simulink model "ThdRwLtStCalib"  (R2024b)
settings: Solver=FixedStepDiscrete  StartTime=0.0  StopTime=10.0  FixedStep=0.01  RelTol=1e-3
model workspace (MAT data in the model file):
  KeSMSwAcsMd6ThdRwLtStBkReclnUpwdDnwdPosMax_Val = Simulink.Parameter
  KeSMSwAcsMd6ThdRwLtStBkReclnUpwdDnwdPosMax_Val.Value = 0
  KeSMSwAcsMd6ThdRwLtStBkReclnUpwdDnwdPosMax_Val.Complexity = 'real'
  KeSMSwAcsMd6ThdRwLtStBkReclnUpwdDnwdPosMax_Val.Dimensions = [1 1]
  KeSMSwAcsMd6ThdRwLtStBkReclnUpwdDnwdPosMax_Val.DataType = 'uint16'
  KeSMSwAcsMd6ThdRwLtStBkReclnUpwdDnwdPosMin_Val = Simulink.Parameter
  KeSMSwAcsMd6ThdRwLtStBkReclnUpwdDnwdPosMin_Val.Value = 0
  KeSMSwAcsMd6ThdRwLtStBkReclnUpwdDnwdPosMin_Val.Complexity = 'real'
  KeSMSwAcsMd6ThdRwLtStBkReclnUpwdDnwdPosMin_Val.Dimensions = [1 1]
  KeSMSwAcsMd6ThdRwLtStBkReclnUpwdDnwdPosMin_Val.DataType = 'uint16'
  KeSMSwAcsMd6ThdRwLtStBkReclnUpwdDnwdPos_Val = Simulink.Parameter
  KeSMSwAcsMd6ThdRwLtStBkReclnUpwdDnwdPos_Val.Value = 0
  KeSMSwAcsMd6ThdRwLtStBkReclnUpwdDnwdPos_Val.Complexity = 'real'
  KeSMSwAcsMd6ThdRwLtStBkReclnUpwdDnwdPos_Val.Dimensions = [1 1]
  KeSMSwAcsMd6ThdRwLtStBkReclnUpwdDnwdPos_Val.DataType = 'uint16'
  KeSMSwAcsMd6ThdRwLtStCshnFldUpwdDnwdPosMax_Val = Simulink.Parameter
  KeSMSwAcsMd6ThdRwLtStCshnFldUpwdDnwdPosMax_Val.Value = 0
  KeSMSwAcsMd6ThdRwLtStCshnFldUpwdDnwdPosMax_Val.Complexity = 'real'
  KeSMSwAcsMd6ThdRwLtStCshnFldUpwdDnwdPosMax_Val.Dimensions = [1 1]
  KeSMSwAcsMd6ThdRwLtStCshnFldUpwdDnwdPosMax_Val.DataType = 'uint16'
  KeSMSwAcsMd6ThdRwLtStCshnFldUpwdDnwdPosMin_Val = Simulink.Parameter
  KeSMSwAcsMd6ThdRwLtStCshnFldUpwdDnwdPosMin_Val.Value = 0
  KeSMSwAcsMd6ThdRwLtStCshnFldUpwdDnwdPosMin_Val.Complexity = 'real'
  KeSMSwAcsMd6ThdRwLtStCshnFldUpwdDnwdPosMin_Val.Dimensions = [1 1]
  KeSMSwAcsMd6ThdRwLtStCshnFldUpwdDnwdPosMin_Val.DataType = 'uint16'
  KeSMSwAcsMd6ThdRwLtStCshnFldUpwdDnwdPos_Val = Simulink.Parameter
  KeSMSwAcsMd6ThdRwLtStCshnFldUpwdDnwdPos_Val.Value = 0
  KeSMSwAcsMd6ThdRwLtStCshnFldUpwdDnwdPos_Val.Complexity = 'real'
  KeSMSwAcsMd6ThdRwLtStCshnFldUpwdDnwdPos_Val.Dimensions = [1 1]
  KeSMSwAcsMd6ThdRwLtStCshnFldUpwdDnwdPos_Val.DataType = 'uint16'
  KeSMSwAcsMd6ThdRwLtStFrwdBkwdPosMax_Val = Simulink.Parameter
  KeSMSwAcsMd6ThdRwLtStFrwdBkwdPosMax_Val.Value = 0
  KeSMSwAcsMd6ThdRwLtStFrwdBkwdPosMax_Val.Complexity = 'real'
  KeSMSwAcsMd6ThdRwLtStFrwdBkwdPosMax_Val.Dimensions = [1 1]
  KeSMSwAcsMd6ThdRwLtStFrwdBkwdPosMax_Val.DataType = 'uint16'
  KeSMSwAcsMd6ThdRwLtStFrwdBkwdPosMin_Val = Simulink.Parameter
  KeSMSwAcsMd6ThdRwLtStFrwdBkwdPosMin_Val.Value = 0
  KeSMSwAcsMd6ThdRwLtStFrwdBkwdPosMin_Val.Complexity = 'real'
  KeSMSwAcsMd6ThdRwLtStFrwdBkwdPosMin_Val.Dimensions = [1 1]
  KeSMSwAcsMd6ThdRwLtStFrwdBkwdPosMin_Val.DataType = 'uint16'
  KeSMSwAcsMd6ThdRwLtStFrwdBkwdPos_Val = Simulink.Parameter
  KeSMSwAcsMd6ThdRwLtStFrwdBkwdPos_Val.Value = 0
  KeSMSwAcsMd6ThdRwLtStFrwdBkwdPos_Val.Complexity = 'real'
  KeSMSwAcsMd6ThdRwLtStFrwdBkwdPos_Val.Dimensions = [1 1]
  KeSMSwAcsMd6ThdRwLtStFrwdBkwdPos_Val.DataType = 'uint16'
undefined symbols (not defined in the file or in its folder): KeSMSw6sAcsEntryThdRwLtStBkReclnUpwdDnwdPos_Val, KeSMSw6sAcsEntryThdRwLtStBkReclnUpwdDnwdPosMax_Val, KeSMSw6sAcsEntryThdRwLtStBkReclnUpwdDnwdPosMin_Val, KeSMSw6sAcsEntryThdRwLtStCshnFldUpwdDnwdPos_Val, KeSMSw6sAcsEntryThdRwLtStCshnFldUpwdDnwdPosMax_Val, KeSMSw6sAcsEntryThdRwLtStCshnFldUpwdDnwdPosMin_Val, KeSMSw6sAcsEntryThdRwLtStFrwdBkwdPos_Val, KeSMSw6sAcsEntryThdRwLtStFrwdBkwdPosMax_Val, KeSMSw6sAcsEntryThdRwLtStFrwdBkwdPosMin_Val, KeSMSw6SAcsMd56ThdRwLtStBkReclnUpwdDnwdPos_Val, KeSMSw6SAcsMd56ThdRwLtStBkReclnUpwdDnwdPosMax_Val, KeSMSw6SAcsMd56ThdRwLtStBkReclnUpwdDnwdPosMin_Val, KeSMSw6SAcsMd56ThdRwLtStFrwdBkwdPos_Val, KeSMSw6SAcsMd56ThdRwLtStFrwdBkwdPosMax_Val, KeSMSw6SAcsMd56ThdRwLtStFrwdBkwdPosMin_Val, KeSMSw6sFamilyLMdThdRwLtStFrwdBkwdPos_Val, KeSMSw6sFamilyLMdThdRwLtStFrwdBkwdPosMax_Val, KeSMSw6sFamilyLMdThdRwLtStFrwdBkwdPosMin_Val, KeSMSw6sFamilyMdThdRwLtStFrwdBkwdPos_Val, KeSMSw6sFamilyMdThdRwLtStFrwdBkwdPosMax_Val, KeSMSw6sFamilyMdThdRwLtStFrwdBkwdPosMin_Val, KeSMSw6sLugThdRwLtStBkReclnUpwdDnwdPos_Val, KeSMSw6sLugThdRwLtStBkReclnUpwdDnwdPosMax_Val, KeSMSw6sLugThdRwLtStBkReclnUpwdDnwdPosMin_Val, KeSMSw6sLugThdRwLtStCshnFldUpwdDnwdPos_Val, KeSMSw6sLugThdRwLtStCshnFldUpwdDnwdPosMax_Val, KeSMSw6sLugThdRwLtStCshnFldUpwdDnwdPosMin_Val, KeSMSw6sVIPThdRwLtStBkReclnUpwdDnwdPos_Val, KeSMSw6sVIPThdRwLtStBkReclnUpwdDnwdPosMax_Val, KeSMSw6sVIPThdRwLtStBkReclnUpwdDnwdPosMin_Val, KeSMSw6sVIPThdRwLtStFrwdBkwdPos_Val, KeSMSw6sVIPThdRwLtStFrwdBkwdPosMax_Val, KeSMSw6sVIPThdRwLtStFrwdBkwdPosMin_Val, KeSMSwAcsEntryThdRwLtStBkReclnUpwdDnwdPos_Val, KeSMSwAcsEntryThdRwLtStBkReclnUpwdDnwdPosMax_Val, KeSMSwAcsEntryThdRwLtStBkReclnUpwdDnwdPosMin_Val, KeSMSwAcsEntryThdRwLtStCshnFldUpwdDnwdPos_Val, KeSMSwAcsEntryThdRwLtStCshnFldUpwdDnwdPosMax_Val, KeSMSwAcsEntryThdRwLtStCshnFldUpwdDnwdPosMin_Val, KeSMSwAcsEntryThdRwLtStFrwdBkwdPos_Val, KeSMSwAcsEntryThdRwLtStFrwdBkwdPosMax_Val, KeSMSwAcsEntryThdRwLtStFrwdBkwdPosMin_Val, KeSMSwAcsMd32ThdRwLtBkReclnUpwdDnwdPos_Val, KeSMSwAcsMd32ThdRwLtBkReclnUpwdDnwdPosMax_Val, KeSMSwAcsMd32ThdRwLtBkReclnUpwdDnwdPosMin_Val, KeSMSwAcsMd32ThdRwLtFldUpwdDnwdPos_Val, KeSMSwAcsMd32ThdRwLtFldUpwdDnwdPosMax_Val, KeSMSwAcsMd32ThdRwLtFldUpwdDnwdPosMin_Val, KeSMSwAcsMd56ThdRwLtStBkReclnUpwdDnwdPos_Val, KeSMSwAcsMd56ThdRwLtStBkReclnUpwdDnwdPosMax_Val, KeSMSwAcsMd56ThdRwLtStBkReclnUpwdDnwdPosMin_Val, KeSMSwAcsMd56ThdRwLtStCshnFldUpwdDnwdPos_Val, KeSMSwAcsMd56ThdRwLtStCshnFldUpwdDnwdPosMax_Val, KeSMSwAcsMd56ThdRwLtStCshnFldUpwdDnwdPosMin_Val, KeSMSwAcsMd56ThdRwLtStFrwdBkwdPos_Val, KeSMSwAcsMd56ThdRwLtStFrwdBkwdPosMax_Val, KeSMSwAcsMd56ThdRwLtStFrwdBkwdPosMin_Val, KeSMSwAcsMd57ThdRwLtStBkReclnUpwdDnwdPos_Val, KeSMSwAcsMd57ThdRwLtStBkReclnUpwdDnwdPosMax_Val, KeSMSwAcsMd57ThdRwLtStBkReclnUpwdDnwdPosMin_Val ... (+28)
libraries: TrgtPosSelcLib x20
(part 1 of 2)
settings Model: ParameterArgumentNames=KeSMSwAcsMd6ThdRwLtStBkReclnUpwdDnwdPosMax_Val,KeSMSwAcsMd6ThdRwLtStBkReclnUpwdDnwdPosMin_Val,KeSMSwAcsMd6ThdRwLtStBkReclnUpwdDnwdPos_Val,KeSMSwAcsMd6ThdRwLtStCshnFldUpwdDnwdPosMax_Val,KeSMSwAcsMd6ThdRwLtStCshnFldUpwdDnwdPosMin_Val,KeSMSwAcsMd6ThdRwLtStCshnFldUpwdDnwdPos_Val,KeSMSwAcsMd6ThdRwLtStFrwdBkwdPosMax_Val,KeSMSwAcsMd6ThdRwLtStFrwdBkwdPosMin_Val,KeSMSwAcsMd6ThdRwLtStFrwdBkwdPos_Val  Creator=sn2xws  LastModifiedBy=sn55gm
settings Model: ModifiedHistory=|
  | 增加Md57，Md58标定，增加6sBitMask
  | 2025.3.5 V3.9.0 Bug 998429 LUG模式偶发不会往前移动三排，但是报成功
settings SolverCC: AlgebraicLoopSolver=TrustRegion
settings DataIOCC: SaveFormat=StructureWithTime  ReturnWorkspaceOutputs=off
settings OptimizationCC: DefaultParameterBehavior=Inlined  EnhancedBackFolding=on  PassReuseOutputArgsAs=Individual arguments  ZeroExternalMemoryAtStartup=off  ZeroInternalMemoryAtStartup=off  OptimizeBlockOrder=speed  DifferentSizesBufferReuse=on  OptimizationCustomize=off  EfficientTunableParamExpr=on
settings DebuggingCC: ParameterTunabilityLossMsg=error  UnconnectedInputMsg=warning  UnconnectedOutputMsg=warning  UnconnectedLineMsg=warning  ArithmeticOperatorsInVariantConditions=warning
settings ModelReferenceCC: EnableRefExpFcnMdlSchedulingChecks=on
settings SFSimCC: MATLABDynamicMemAlloc=off  CustomCodeUndefinedFunction=UseInterfaceOnly
settings RTWCC: Description=AUTOSAR  SystemTargetFile=autosar.tlc  GenCodeOnly=on  TemplateMakefile=ert_default_tmf  GenerateReport=on  IncludeHyperlinkInReport=on  LaunchReport=on  DataTypeReplacement=CDataTypesFixedWidth  GenerateTraceInfo=on  GenerateTraceReport=on  GenerateTraceReportSl=on  GenerateTraceReportSf=on  GenerateTraceReportEml=on  GPUComputeCapability=3.5
settings CodeAppCC: ForceParamTrailComments=on  IgnoreCustomStorageClasses=off  OperatorAnnotations=on  SimulinkDataObjDesc=on  SFDataObjDesc=on  InsertBlockDesc=on
settings STFCustomTargetCC: TargetLangStandard=C99 (ISO)  MultiwordLength=256  ParMdlRefBuildCompliant=on  CompOptLevelCompliant=on  IncludeMdlTerminateFcn=off  CombineOutputUpdateFcns=on  SuppressErrorStatus=on  ERTCustomFileBanners=on  SupportNonFinite=off  SupportComplex=off  SupportContinuousTime=off  SupportNonInlinedSFcns=off  RemoveResetFunc=on  MATLABClassNameForMDSCustomization=Simulink.SoftwareTarget.ERTCustomization  AutosarCompliant=on  UseToolchainInfoCompliant=on  LookupTableObjectStructAxisOrder=2,1,3,4,...  LUTObjectStructOrderEvenSpacing=Size,Table,Breakpoints  SystemTargetFile=autosar.tlc
settings ERTTargetCC: TargetLangStandard=C99 (ISO)  ConcurrentExecutionCompliant=off  IncludeMdlTerminateFcn=off  SuppressErrorStatus=on  SupportNonFinite=off  SupportComplex=off  ModelStepFunctionPrototypeControlCompliant=off  CPPClassGenCompliant=off  AutosarCompliant=on  LookupTableObjectStructAxisOrder=2,1,3,4,...  LUTObjectStructOrderEvenSpacing=Size,Table,Breakpoints  ERTCustomFileTemplate=example_file_process.tlc  ERTFilePackagingFormat=Compact  BooleanTrueId=TRUE  BooleanFalseId=FALSE  DynamicArrayContainerType=coder::array

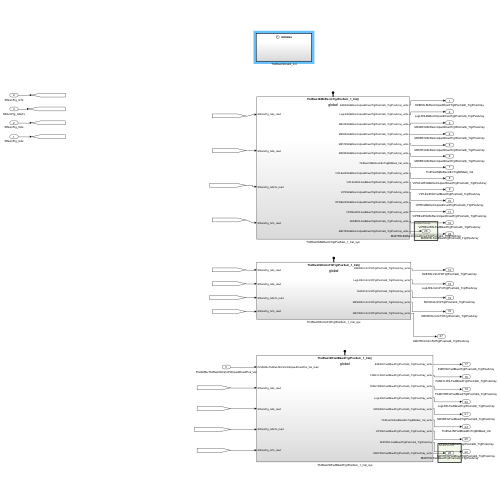
[thumbnail: Simulink's stored preview of the top-level diagram]
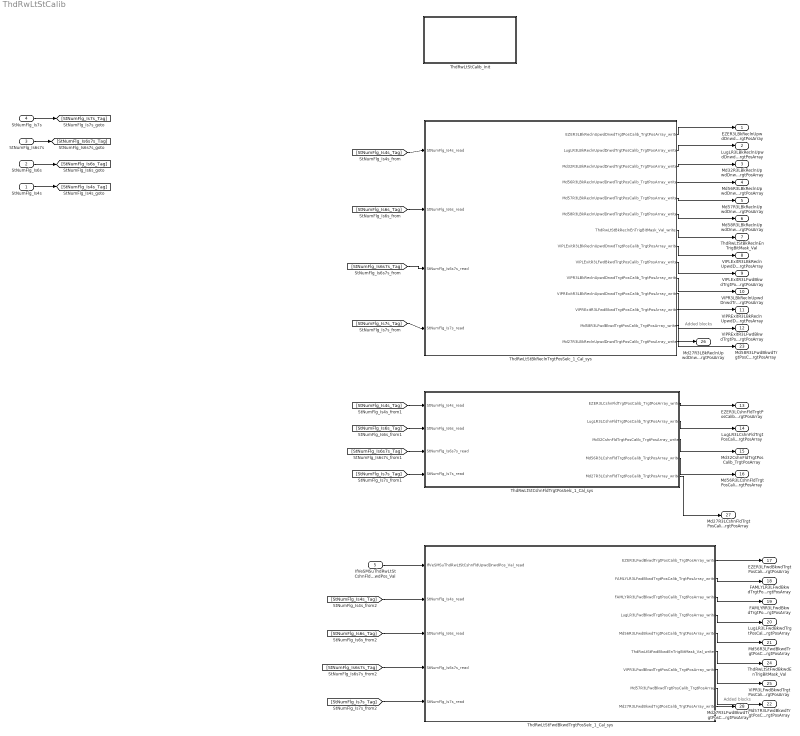
== system ThdRwLtStCalib ==
  note: Added blocks
  note: Added blocks
  StNumFlg_Is4s : Inport  OutDataTypeStr=boolean  PortDimensions=1
  StNumFlg_Is6s : Inport  Port=2  OutDataTypeStr=boolean  PortDimensions=1
  StNumFlg_Is6s7s : Inport  Port=3  OutDataTypeStr=boolean  PortDimensions=1
  StNumFlg_Is7s : Inport  Port=4  OutDataTypeStr=boolean  PortDimensions=1
  IfVeSMSuThdRwLtStCshnFldUpwdDnwdPos_Val : Inport  Port=5  OutDataTypeStr=uint16  PortDimensions=1
  ThdRwLtStBkReclnTrgtPosSelc_1_Cal_sys : Subsystem
  ThdRwLtStCalib_Init : Subsystem
  ThdRwLtStCshnFldTrgtPosSelc_1_Cal_sys : Subsystem
  ThdRwLtStFwdBkwdTrgtPosSelc_1_Cal_sys : Subsystem
  EZER3LBkReclnUpwdDnwdTrgtPosCalib_TrgtPosArray : Outport  Description=|  OutDataTypeStr=uint16  PortDimensions=3  VectorParamsAs1DForOutWhenUnconnected=off
      | 0:Pos
      | 1:Max
      | 2:Min
  LugLR3LBkReclnUpwdDnwdTrgtPosCalib_TrgtPosArray : Outport  Description=|  Port=2  OutDataTypeStr=uint16  PortDimensions=3  VectorParamsAs1DForOutWhenUnconnected=off
      | 0:Pos
      | 1:Max
      | 2:Min
  Md32R3LBkReclnUpwdDnwdTrgtPosCalib_TrgtPosArray : Outport  Description=|  Port=3  OutDataTypeStr=uint16  PortDimensions=3  VectorParamsAs1DForOutWhenUnconnected=off
      | 0:Pos
      | 1:Max
      | 2:Min
  Md56R3LBkReclnUpwdDnwdTrgtPosCalib_TrgtPosArray : Outport  Description=|  Port=4  OutDataTypeStr=uint16  PortDimensions=3  VectorParamsAs1DForOutWhenUnconnected=off
      | 0:Pos
      | 1:Max
      | 2:Min
  Md57R3LBkReclnUpwdDnwdTrgtPosCalib_TrgtPosArray : Outport  Description=|  Port=5  OutDataTypeStr=uint16  PortDimensions=3  VectorParamsAs1DForOutWhenUnconnected=off
      | 0:Pos
      | 1:Max
      | 2:Min
  Md58R3LBkReclnUpwdDnwdTrgtPosCalib_TrgtPosArray : Outport  Description=|  Port=6  OutDataTypeStr=uint16  PortDimensions=3  VectorParamsAs1DForOutWhenUnconnected=off
      | 0:Pos
      | 1:Max
      | 2:Min
  ThdRwLtStBkReclnEnTrigBitMask_Val : Outport  Port=7  OutDataTypeStr=uint32  PortDimensions=1  VectorParamsAs1DForOutWhenUnconnected=off
  VIPLExitR3LBkReclnUpwdDnwdTrgtPosCalib_TrgtPosArray : Outport  Description=|  Port=8  OutDataTypeStr=uint16  PortDimensions=3  VectorParamsAs1DForOutWhenUnconnected=off
      | 0:Pos
      | 1:Max
      | 2:Min
  VIPLExitR3LFwdBkwdTrgtPosCalib_TrgtPosArray : Outport  Description=|  Port=9  OutDataTypeStr=uint16  PortDimensions=3  VectorParamsAs1DForOutWhenUnconnected=off
      | 0:Pos
      | 1:Max
      | 2:Min
  VIPR3LBkReclnUpwdDnwdTrgtPosCalib_TrgtPosArray : Outport  Description=|  Port=10  OutDataTypeStr=uint16  PortDimensions=3  VectorParamsAs1DForOutWhenUnconnected=off
      | 0:Pos
      | 1:Max
      | 2:Min
  VIPRExitR3LBkReclnUpwdDnwdTrgtPosCalib_TrgtPosArray : Outport  Description=|  Port=11  OutDataTypeStr=uint16  PortDimensions=3  VectorParamsAs1DForOutWhenUnconnected=off
      | 0:Pos
      | 1:Max
      | 2:Min
  VIPRExitR3LFwdBkwdTrgtPosCalib_TrgtPosArray : Outport  Description=|  Port=12  OutDataTypeStr=uint16  PortDimensions=3  VectorParamsAs1DForOutWhenUnconnected=off
      | 0:Pos
      | 1:Max
      | 2:Min
  EZER3LCshnFldTrgtPosCalib_TrgtPosArray : Outport  Description=|  Port=13  OutDataTypeStr=uint16  PortDimensions=3  VectorParamsAs1DForOutWhenUnconnected=off
      | 0:Pos
      | 1:Max
      | 2:Min
  LugLR3LCshnFldTrgtPosCalib_TrgtPosArray : Outport  Description=|  Port=14  OutDataTypeStr=uint16  PortDimensions=3  VectorParamsAs1DForOutWhenUnconnected=off
      | 0:Pos
      | 1:Max
      | 2:Min
  Md32CshnFldTrgtPosCalib_TrgtPosArray : Outport  Description=|  Port=15  OutDataTypeStr=uint16  PortDimensions=3  VectorParamsAs1DForOutWhenUnconnected=off
      | 0:Pos
      | 1:Max
      | 2:Min
  Md56R3LCshnFldTrgtPosCalib_TrgtPosArray : Outport  Description=|  Port=16  OutDataTypeStr=uint16  PortDimensions=3  VectorParamsAs1DForOutWhenUnconnected=off
      | 0:Pos
      | 1:Max
      | 2:Min
  EZER3LFwdBkwdTrgtPosCalib_TrgtPosArray : Outport  Description=|  Port=17  OutDataTypeStr=uint16  PortDimensions=3  VectorParamsAs1DForOutWhenUnconnected=off
      | 0:Pos
      | 1:Max
      | 2:Min
  FAMLYLR3LFwdBkwdTrgtPosCalib_TrgtPosArray : Outport  Description=|  Port=18  OutDataTypeStr=uint16  PortDimensions=3  VectorParamsAs1DForOutWhenUnconnected=off
      | 0:Pos
      | 1:Max
      | 2:Min
  FAMLYRR3LFwdBkwdTrgtPosCalib_TrgtPosArray : Outport  Description=|  Port=19  OutDataTypeStr=uint16  PortDimensions=3  VectorParamsAs1DForOutWhenUnconnected=off
      | 0:Pos
      | 1:Max
      | 2:Min
  LugLR3LFwdBkwdTrgtPosCalib_TrgtPosArray : Outport  Description=|  Port=20  OutDataTypeStr=uint16  PortDimensions=3  VectorParamsAs1DForOutWhenUnconnected=off
      | 0:Pos
      | 1:Max
      | 2:Min
  Md56R3LFwdBkwdTrgtPosCalib_TrgtPosArray : Outport  Description=|  Port=21  OutDataTypeStr=uint16  PortDimensions=3  VectorParamsAs1DForOutWhenUnconnected=off
      | 0:Pos
      | 1:Max
      | 2:Min
  Md57R3LFwdBkwdTrgtPosCalib_TrgtPosArray : Outport  Description=|  Port=22  OutDataTypeStr=uint16  PortDimensions=3  VectorParamsAs1DForOutWhenUnconnected=off
      | 0:Pos
      | 1:Max
      | 2:Min
  Md58R3LFwdBkwdTrgtPosCalib_TrgtPosArray : Outport  Description=|  Port=23  OutDataTypeStr=uint16  PortDimensions=3  VectorParamsAs1DForOutWhenUnconnected=off
      | 0:Pos
      | 1:Max
      | 2:Min
  ThdRwLtStFwdBkwdEnTrigBitMask_Val : Outport  Port=24  OutDataTypeStr=uint32  PortDimensions=1  VectorParamsAs1DForOutWhenUnconnected=off
  VIPR3LFwdBkwdTrgtPosCalib_TrgtPosArray : Outport  Description=|  Port=25  OutDataTypeStr=uint16  PortDimensions=3  VectorParamsAs1DForOutWhenUnconnected=off
      | 0:Pos
      | 1:Max
      | 2:Min
  Md27R3LBkReclnUpwdDnwdTrgtPosCalib_TrgtPosArray : Outport  Description=|  Port=26  OutDataTypeStr=uint16  PortDimensions=3  VectorParamsAs1DForOutWhenUnconnected=off
      | 0:Pos
      | 1:Max
      | 2:Min
  Md27R3LCshnFldTrgtPosCalib_TrgtPosArray : Outport  Description=|  Port=27  OutDataTypeStr=uint16  PortDimensions=3  VectorParamsAs1DForOutWhenUnconnected=off
      | 0:Pos
      | 1:Max
      | 2:Min
  Md27R3LFwdBkwdTrgtPosCalib_TrgtPosArray : Outport  Description=|  Port=28  OutDataTypeStr=uint16  PortDimensions=3  VectorParamsAs1DForOutWhenUnconnected=off
      | 0:Pos
      | 1:Max
      | 2:Min
  wires:
  ThdRwLtStBkReclnTrgtPosSelc_1_Cal_sys/1(EZER3LBkReclnUpwdDnwdTrgtPosCalib_TrgtPosArray_write) -> EZER3LBkReclnUpwdDnwdTrgtPosCalib_TrgtPosArray/1
  ThdRwLtStBkReclnTrgtPosSelc_1_Cal_sys/2(LugLR3LBkReclnUpwdDnwdTrgtPosCalib_TrgtPosArray_write) -> LugLR3LBkReclnUpwdDnwdTrgtPosCalib_TrgtPosArray/1
  ThdRwLtStBkReclnTrgtPosSelc_1_Cal_sys/3(Md32R3LBkReclnUpwdDnwdTrgtPosCalib_TrgtPosArray_write) -> Md32R3LBkReclnUpwdDnwdTrgtPosCalib_TrgtPosArray/1
  ThdRwLtStBkReclnTrgtPosSelc_1_Cal_sys/4(Md56R3LBkReclnUpwdDnwdTrgtPosCalib_TrgtPosArray_write) -> Md56R3LBkReclnUpwdDnwdTrgtPosCalib_TrgtPosArray/1
  ThdRwLtStBkReclnTrgtPosSelc_1_Cal_sys/5(Md57R3LBkReclnUpwdDnwdTrgtPosCalib_TrgtPosArray_write) -> Md57R3LBkReclnUpwdDnwdTrgtPosCalib_TrgtPosArray/1
  ThdRwLtStBkReclnTrgtPosSelc_1_Cal_sys/6(Md58R3LBkReclnUpwdDnwdTrgtPosCalib_TrgtPosArray_write) -> Md58R3LBkReclnUpwdDnwdTrgtPosCalib_TrgtPosArray/1
  ThdRwLtStBkReclnTrgtPosSelc_1_Cal_sys/7(ThdRwLtStBkReclnEnTrigBitMask_Val_write) -> ThdRwLtStBkReclnEnTrigBitMask_Val/1
  ThdRwLtStBkReclnTrgtPosSelc_1_Cal_sys/8(VIPLExitR3LBkReclnUpwdDnwdTrgtPosCalib_TrgtPosArray_write) -> VIPLExitR3LBkReclnUpwdDnwdTrgtPosCalib_TrgtPosArray/1
  ThdRwLtStBkReclnTrgtPosSelc_1_Cal_sys/9(VIPLExitR3LFwdBkwdTrgtPosCalib_TrgtPosArray_write) -> VIPLExitR3LFwdBkwdTrgtPosCalib_TrgtPosArray/1
  ThdRwLtStBkReclnTrgtPosSelc_1_Cal_sys/10(VIPR3LBkReclnUpwdDnwdTrgtPosCalib_TrgtPosArray_write) -> VIPR3LBkReclnUpwdDnwdTrgtPosCalib_TrgtPosArray/1
  ThdRwLtStBkReclnTrgtPosSelc_1_Cal_sys/11(VIPRExitR3LBkReclnUpwdDnwdTrgtPosCalib_TrgtPosArray_write) -> VIPRExitR3LBkReclnUpwdDnwdTrgtPosCalib_TrgtPosArray/1
  ThdRwLtStBkReclnTrgtPosSelc_1_Cal_sys/12(VIPRExitR3LFwdBkwdTrgtPosCalib_TrgtPosArray_write) -> VIPRExitR3LFwdBkwdTrgtPosCalib_TrgtPosArray/1
  ThdRwLtStCshnFldTrgtPosSelc_1_Cal_sys/1(EZER3LCshnFldTrgtPosCalib_TrgtPosArray_write) -> EZER3LCshnFldTrgtPosCalib_TrgtPosArray/1
  ThdRwLtStCshnFldTrgtPosSelc_1_Cal_sys/2(LugLR3LCshnFldTrgtPosCalib_TrgtPosArray_write) -> LugLR3LCshnFldTrgtPosCalib_TrgtPosArray/1
  ThdRwLtStCshnFldTrgtPosSelc_1_Cal_sys/3(Md32CshnFldTrgtPosCalib_TrgtPosArray_write) -> Md32CshnFldTrgtPosCalib_TrgtPosArray/1
  ThdRwLtStCshnFldTrgtPosSelc_1_Cal_sys/4(Md56R3LCshnFldTrgtPosCalib_TrgtPosArray_write) -> Md56R3LCshnFldTrgtPosCalib_TrgtPosArray/1
  IfVeSMSuThdRwLtStCshnFldUpwdDnwdPos_Val/1 -> ThdRwLtStFwdBkwdTrgtPosSelc_1_Cal_sys/1(IfVeSMSuThdRwLtStCshnFldUpwdDnwdPos_Val_read)
  ThdRwLtStFwdBkwdTrgtPosSelc_1_Cal_sys/1(EZER3LFwdBkwdTrgtPosCalib_TrgtPosArray_write) -> EZER3LFwdBkwdTrgtPosCalib_TrgtPosArray/1
  ThdRwLtStFwdBkwdTrgtPosSelc_1_Cal_sys/2(FAMLYLR3LFwdBkwdTrgtPosCalib_TrgtPosArray_write) -> FAMLYLR3LFwdBkwdTrgtPosCalib_TrgtPosArray/1
  ThdRwLtStFwdBkwdTrgtPosSelc_1_Cal_sys/3(FAMLYRR3LFwdBkwdTrgtPosCalib_TrgtPosArray_write) -> FAMLYRR3LFwdBkwdTrgtPosCalib_TrgtPosArray/1
  ThdRwLtStFwdBkwdTrgtPosSelc_1_Cal_sys/4(LugLR3LFwdBkwdTrgtPosCalib_TrgtPosArray_write) -> LugLR3LFwdBkwdTrgtPosCalib_TrgtPosArray/1
  ThdRwLtStFwdBkwdTrgtPosSelc_1_Cal_sys/5(Md56R3LFwdBkwdTrgtPosCalib_TrgtPosArray_write) -> Md56R3LFwdBkwdTrgtPosCalib_TrgtPosArray/1
  ThdRwLtStFwdBkwdTrgtPosSelc_1_Cal_sys/8(Md57R3LFwdBkwdTrgtPosCalib_TrgtPosArray) -> Md57R3LFwdBkwdTrgtPosCalib_TrgtPosArray/1
  ThdRwLtStFwdBkwdTrgtPosSelc_1_Cal_sys/6(ThdRwLtStFwdBkwdEnTrigBitMask_Val_write) -> ThdRwLtStFwdBkwdEnTrigBitMask_Val/1
  ThdRwLtStFwdBkwdTrgtPosSelc_1_Cal_sys/7(VIPR3LFwdBkwdTrgtPosCalib_TrgtPosArray_write) -> VIPR3LFwdBkwdTrgtPosCalib_TrgtPosArray/1
  StNumFlg_Is7s/1 -> [StNumFlg_Is7s_Tag]
  [StNumFlg_Is7s_Tag] -> ThdRwLtStBkReclnTrgtPosSelc_1_Cal_sys/4(StNumFlg_Is7s_read)
  [StNumFlg_Is7s_Tag] -> ThdRwLtStCshnFldTrgtPosSelc_1_Cal_sys/4(StNumFlg_Is7s_read)
  [StNumFlg_Is7s_Tag] -> ThdRwLtStFwdBkwdTrgtPosSelc_1_Cal_sys/5(StNumFlg_Is7s_read)
  StNumFlg_Is6s7s/1 -> [StNumFlg_Is6s7s_Tag]
  [StNumFlg_Is6s7s_Tag] -> ThdRwLtStBkReclnTrgtPosSelc_1_Cal_sys/3(StNumFlg_Is6s7s_read)
  [StNumFlg_Is6s7s_Tag] -> ThdRwLtStCshnFldTrgtPosSelc_1_Cal_sys/3(StNumFlg_Is6s7s_read)
  [StNumFlg_Is6s7s_Tag] -> ThdRwLtStFwdBkwdTrgtPosSelc_1_Cal_sys/4(StNumFlg_Is6s7s_read)
  StNumFlg_Is6s/1 -> [StNumFlg_Is6s_Tag]
  [StNumFlg_Is6s_Tag] -> ThdRwLtStBkReclnTrgtPosSelc_1_Cal_sys/2(StNumFlg_Is6s_read)
  [StNumFlg_Is6s_Tag] -> ThdRwLtStCshnFldTrgtPosSelc_1_Cal_sys/2(StNumFlg_Is6s_read)
  [StNumFlg_Is6s_Tag] -> ThdRwLtStFwdBkwdTrgtPosSelc_1_Cal_sys/3(StNumFlg_Is6s_read)
  StNumFlg_Is4s/1 -> [StNumFlg_Is4s_Tag]
  [StNumFlg_Is4s_Tag] -> ThdRwLtStBkReclnTrgtPosSelc_1_Cal_sys/1(StNumFlg_Is4s_read)
  [StNumFlg_Is4s_Tag] -> ThdRwLtStCshnFldTrgtPosSelc_1_Cal_sys/1(StNumFlg_Is4s_read)
  [StNumFlg_Is4s_Tag] -> ThdRwLtStFwdBkwdTrgtPosSelc_1_Cal_sys/2(StNumFlg_Is4s_read)
  ThdRwLtStBkReclnTrgtPosSelc_1_Cal_sys/13(Md58R3LFwdBkwdTrgtPosCalib_TrgtPosArray_write) -> Md58R3LFwdBkwdTrgtPosCalib_TrgtPosArray/1
  ThdRwLtStBkReclnTrgtPosSelc_1_Cal_sys/14(Md27R3LBkReclnUpwdDnwdTrgtPosCalib_TrgtPosArray_write) -> Md27R3LBkReclnUpwdDnwdTrgtPosCalib_TrgtPosArray/1
  ThdRwLtStCshnFldTrgtPosSelc_1_Cal_sys/5(Md27R3LCshnFldTrgtPosCalib_TrgtPosArray_write) -> Md27R3LCshnFldTrgtPosCalib_TrgtPosArray/1
  ThdRwLtStFwdBkwdTrgtPosSelc_1_Cal_sys/9(Md27R3LFwdBkwdTrgtPosCalib_TrgtPosArray_write) -> Md27R3LFwdBkwdTrgtPosCalib_TrgtPosArray/1

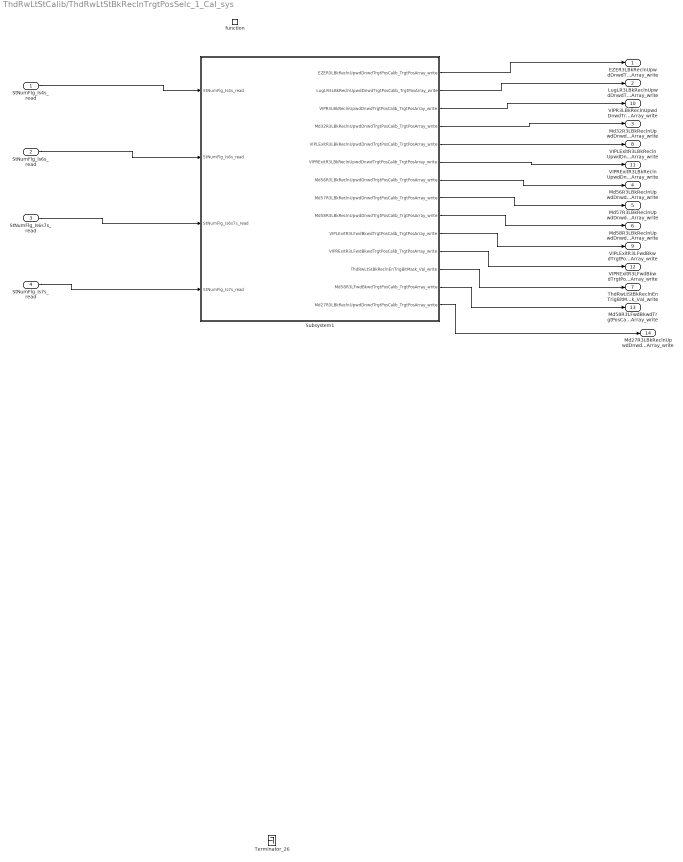
== system ThdRwLtStCalib/ThdRwLtStBkReclnTrgtPosSelc_1_Cal_sys ==
  StNumFlg_Is4s_read : Inport
  StNumFlg_Is6s_read : Inport  Port=2
  StNumFlg_Is6s7s_read : Inport  Port=3
  StNumFlg_Is7s_read : Inport  Port=4
  function : TriggerPort  TriggerType=function-call  IsSimulinkFunction=on  FunctionName=ThdRwLtStBkReclnTrgtPosSelc_1_Cal  VariantControl=(inherit)
  Subsystem1 : Subsystem
  Terminator_26 : Terminator
  EZER3LBkReclnUpwdDnwdTrgtPosCalib_TrgtPosArray_write : Outport  VectorParamsAs1DForOutWhenUnconnected=off
  LugLR3LBkReclnUpwdDnwdTrgtPosCalib_TrgtPosArray_write : Outport  Port=2  VectorParamsAs1DForOutWhenUnconnected=off
  Md32R3LBkReclnUpwdDnwdTrgtPosCalib_TrgtPosArray_write : Outport  Port=3  VectorParamsAs1DForOutWhenUnconnected=off
  Md56R3LBkReclnUpwdDnwdTrgtPosCalib_TrgtPosArray_write : Outport  Port=4  VectorParamsAs1DForOutWhenUnconnected=off
  Md57R3LBkReclnUpwdDnwdTrgtPosCalib_TrgtPosArray_write : Outport  Port=5  VectorParamsAs1DForOutWhenUnconnected=off
  Md58R3LBkReclnUpwdDnwdTrgtPosCalib_TrgtPosArray_write : Outport  Port=6  VectorParamsAs1DForOutWhenUnconnected=off
  ThdRwLtStBkReclnEnTrigBitMask_Val_write : Outport  Port=7  VectorParamsAs1DForOutWhenUnconnected=off
  VIPLExitR3LBkReclnUpwdDnwdTrgtPosCalib_TrgtPosArray_write : Outport  Port=8  VectorParamsAs1DForOutWhenUnconnected=off
  VIPLExitR3LFwdBkwdTrgtPosCalib_TrgtPosArray_write : Outport  Port=9  VectorParamsAs1DForOutWhenUnconnected=off
  VIPR3LBkReclnUpwdDnwdTrgtPosCalib_TrgtPosArray_write : Outport  Port=10  VectorParamsAs1DForOutWhenUnconnected=off
  VIPRExitR3LBkReclnUpwdDnwdTrgtPosCalib_TrgtPosArray_write : Outport  Port=11  VectorParamsAs1DForOutWhenUnconnected=off
  VIPRExitR3LFwdBkwdTrgtPosCalib_TrgtPosArray_write : Outport  Port=12  VectorParamsAs1DForOutWhenUnconnected=off
  Md58R3LFwdBkwdTrgtPosCalib_TrgtPosArray_write : Outport  Port=13  VectorParamsAs1DForOutWhenUnconnected=off
  Md27R3LBkReclnUpwdDnwdTrgtPosCalib_TrgtPosArray_write : Outport  Port=14  VectorParamsAs1DForOutWhenUnconnected=off
      settings: EnsureOutportIsVirtual=on
  wires:
  StNumFlg_Is4s_read/1 -> Subsystem1/1(StNumFlg_Is4s_read)
  StNumFlg_Is6s_read/1 -> Subsystem1/2(StNumFlg_Is6s_read)
  StNumFlg_Is6s7s_read/1 -> Subsystem1/3(StNumFlg_Is6s7s_read)
  StNumFlg_Is7s_read/1 -> Subsystem1/4(StNumFlg_Is7s_read)
  Subsystem1/1(EZER3LBkReclnUpwdDnwdTrgtPosCalib_TrgtPosArray_write) -> EZER3LBkReclnUpwdDnwdTrgtPosCalib_TrgtPosArray_write/1
  Subsystem1/2(LugLR3LBkReclnUpwdDnwdTrgtPosCalib_TrgtPosArray_write) -> LugLR3LBkReclnUpwdDnwdTrgtPosCalib_TrgtPosArray_write/1
  Subsystem1/3(VIPR3LBkReclnUpwdDnwdTrgtPosCalib_TrgtPosArray_write) -> VIPR3LBkReclnUpwdDnwdTrgtPosCalib_TrgtPosArray_write/1
  Subsystem1/4(Md32R3LBkReclnUpwdDnwdTrgtPosCalib_TrgtPosArray_write) -> Md32R3LBkReclnUpwdDnwdTrgtPosCalib_TrgtPosArray_write/1
  Subsystem1/5(VIPLExitR3LBkReclnUpwdDnwdTrgtPosCalib_TrgtPosArray_write) -> VIPLExitR3LBkReclnUpwdDnwdTrgtPosCalib_TrgtPosArray_write/1
  Subsystem1/6(VIPRExitR3LBkReclnUpwdDnwdTrgtPosCalib_TrgtPosArray_write) -> VIPRExitR3LBkReclnUpwdDnwdTrgtPosCalib_TrgtPosArray_write/1
  Subsystem1/7(Md56R3LBkReclnUpwdDnwdTrgtPosCalib_TrgtPosArray_write) -> Md56R3LBkReclnUpwdDnwdTrgtPosCalib_TrgtPosArray_write/1
  Subsystem1/8(Md57R3LBkReclnUpwdDnwdTrgtPosCalib_TrgtPosArray_write) -> Md57R3LBkReclnUpwdDnwdTrgtPosCalib_TrgtPosArray_write/1
  Subsystem1/9(Md58R3LBkReclnUpwdDnwdTrgtPosCalib_TrgtPosArray_write) -> Md58R3LBkReclnUpwdDnwdTrgtPosCalib_TrgtPosArray_write/1
  Subsystem1/10(VIPLExitR3LFwdBkwdTrgtPosCalib_TrgtPosArray_write) -> VIPLExitR3LFwdBkwdTrgtPosCalib_TrgtPosArray_write/1
  Subsystem1/11(VIPRExitR3LFwdBkwdTrgtPosCalib_TrgtPosArray_write) -> VIPRExitR3LFwdBkwdTrgtPosCalib_TrgtPosArray_write/1
  Subsystem1/12(ThdRwLtStBkReclnEnTrigBitMask_Val_write) -> ThdRwLtStBkReclnEnTrigBitMask_Val_write/1
  Subsystem1/13(Md58R3LFwdBkwdTrgtPosCalib_TrgtPosArray_write) -> Md58R3LFwdBkwdTrgtPosCalib_TrgtPosArray_write/1
  ? -> Terminator_26/1
  Subsystem1/14(Md27R3LBkReclnUpwdDnwdTrgtPosCalib_TrgtPosArray_write) -> Md27R3LBkReclnUpwdDnwdTrgtPosCalib_TrgtPosArray_write/1

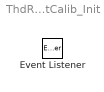
== system ThdRwLtStCalib/ThdRwLtStCalib_Init ==
  Event Listener : EventListener  EventName=reset

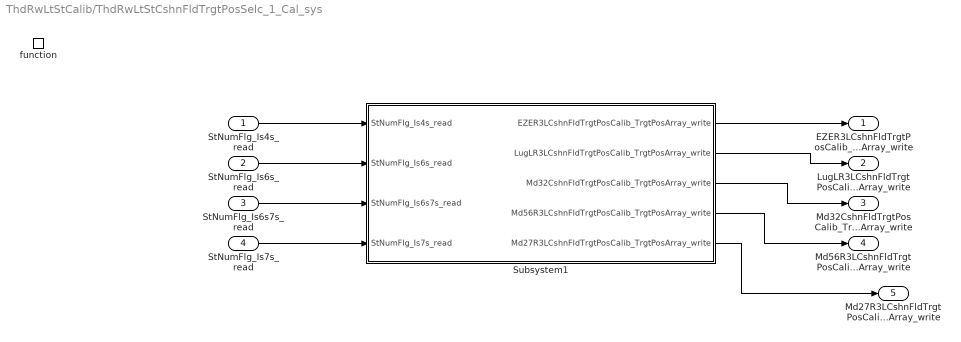
== system ThdRwLtStCalib/ThdRwLtStCshnFldTrgtPosSelc_1_Cal_sys ==
  StNumFlg_Is4s_read : Inport
  StNumFlg_Is6s_read : Inport  Port=2
  StNumFlg_Is6s7s_read : Inport  Port=3
  StNumFlg_Is7s_read : Inport  Port=4
  function : TriggerPort  TriggerType=function-call  IsSimulinkFunction=on  FunctionName=ThdRwLtStCshnFldTrgtPosSelc_1_Cal  VariantControl=(inherit)
  Subsystem1 : Subsystem
  EZER3LCshnFldTrgtPosCalib_TrgtPosArray_write : Outport  VectorParamsAs1DForOutWhenUnconnected=off
  LugLR3LCshnFldTrgtPosCalib_TrgtPosArray_write : Outport  Port=2  VectorParamsAs1DForOutWhenUnconnected=off
  Md32CshnFldTrgtPosCalib_TrgtPosArray_write : Outport  Port=3  VectorParamsAs1DForOutWhenUnconnected=off
  Md56R3LCshnFldTrgtPosCalib_TrgtPosArray_write : Outport  Port=4  VectorParamsAs1DForOutWhenUnconnected=off
  Md27R3LCshnFldTrgtPosCalib_TrgtPosArray_write : Outport  Port=5  VectorParamsAs1DForOutWhenUnconnected=off
      settings: EnsureOutportIsVirtual=on
  wires:
  Subsystem1/4(Md56R3LCshnFldTrgtPosCalib_TrgtPosArray_write) -> Md56R3LCshnFldTrgtPosCalib_TrgtPosArray_write/1
  Subsystem1/3(Md32CshnFldTrgtPosCalib_TrgtPosArray_write) -> Md32CshnFldTrgtPosCalib_TrgtPosArray_write/1
  Subsystem1/2(LugLR3LCshnFldTrgtPosCalib_TrgtPosArray_write) -> LugLR3LCshnFldTrgtPosCalib_TrgtPosArray_write/1
  Subsystem1/1(EZER3LCshnFldTrgtPosCalib_TrgtPosArray_write) -> EZER3LCshnFldTrgtPosCalib_TrgtPosArray_write/1
  StNumFlg_Is4s_read/1 -> Subsystem1/1(StNumFlg_Is4s_read)
  StNumFlg_Is6s_read/1 -> Subsystem1/2(StNumFlg_Is6s_read)
  StNumFlg_Is6s7s_read/1 -> Subsystem1/3(StNumFlg_Is6s7s_read)
  StNumFlg_Is7s_read/1 -> Subsystem1/4(StNumFlg_Is7s_read)
  Subsystem1/5(Md27R3LCshnFldTrgtPosCalib_TrgtPosArray_write) -> Md27R3LCshnFldTrgtPosCalib_TrgtPosArray_write/1

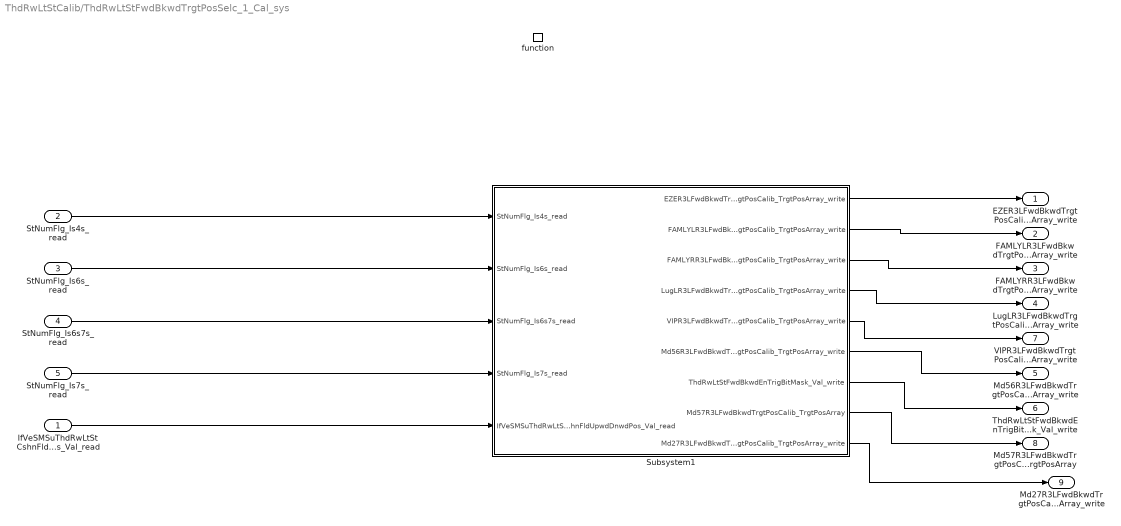
== system ThdRwLtStCalib/ThdRwLtStFwdBkwdTrgtPosSelc_1_Cal_sys ==
  IfVeSMSuThdRwLtStCshnFldUpwdDnwdPos_Val_read : Inport
  StNumFlg_Is4s_read : Inport  Port=2
  StNumFlg_Is6s_read : Inport  Port=3
  StNumFlg_Is6s7s_read : Inport  Port=4
  StNumFlg_Is7s_read : Inport  Port=5
  function : TriggerPort  TriggerType=function-call  IsSimulinkFunction=on  FunctionName=ThdRwLtStFwdBkwdTrgtPosSelc_1_Cal  VariantControl=(inherit)
  Subsystem1 : Subsystem
  EZER3LFwdBkwdTrgtPosCalib_TrgtPosArray_write : Outport  VectorParamsAs1DForOutWhenUnconnected=off
      settings: EnsureOutportIsVirtual=on
  FAMLYLR3LFwdBkwdTrgtPosCalib_TrgtPosArray_write : Outport  Port=2  VectorParamsAs1DForOutWhenUnconnected=off
      settings: EnsureOutportIsVirtual=on
  FAMLYRR3LFwdBkwdTrgtPosCalib_TrgtPosArray_write : Outport  Port=3  VectorParamsAs1DForOutWhenUnconnected=off
      settings: EnsureOutportIsVirtual=on
  LugLR3LFwdBkwdTrgtPosCalib_TrgtPosArray_write : Outport  Port=4  VectorParamsAs1DForOutWhenUnconnected=off
      settings: EnsureOutportIsVirtual=on
  Md56R3LFwdBkwdTrgtPosCalib_TrgtPosArray_write : Outport  Port=5  VectorParamsAs1DForOutWhenUnconnected=off
      settings: EnsureOutportIsVirtual=on
  ThdRwLtStFwdBkwdEnTrigBitMask_Val_write : Outport  Port=6  VectorParamsAs1DForOutWhenUnconnected=off
      settings: EnsureOutportIsVirtual=on
  VIPR3LFwdBkwdTrgtPosCalib_TrgtPosArray_write : Outport  Port=7  VectorParamsAs1DForOutWhenUnconnected=off
      settings: EnsureOutportIsVirtual=on
  Md57R3LFwdBkwdTrgtPosCalib_TrgtPosArray : Outport  Description=|  Port=8  OutDataTypeStr=uint16  PortDimensions=3  VectorParamsAs1DForOutWhenUnconnected=off
      | 0:Pos
      | 1:Max
      | 2:Min
  Md27R3LFwdBkwdTrgtPosCalib_TrgtPosArray_write : Outport  Port=9  VectorParamsAs1DForOutWhenUnconnected=off
      settings: EnsureOutportIsVirtual=on
  wires:
  StNumFlg_Is4s_read/1 -> Subsystem1/1(StNumFlg_Is4s_read)
  StNumFlg_Is6s_read/1 -> Subsystem1/2(StNumFlg_Is6s_read)
  StNumFlg_Is6s7s_read/1 -> Subsystem1/3(StNumFlg_Is6s7s_read)
  StNumFlg_Is7s_read/1 -> Subsystem1/4(StNumFlg_Is7s_read)
  IfVeSMSuThdRwLtStCshnFldUpwdDnwdPos_Val_read/1 -> Subsystem1/5(IfVeSMSuThdRwLtStCshnFldUpwdDnwdPos_Val_read)
  Subsystem1/1(EZER3LFwdBkwdTrgtPosCalib_TrgtPosArray_write) -> EZER3LFwdBkwdTrgtPosCalib_TrgtPosArray_write/1
  Subsystem1/2(FAMLYLR3LFwdBkwdTrgtPosCalib_TrgtPosArray_write) -> FAMLYLR3LFwdBkwdTrgtPosCalib_TrgtPosArray_write/1
  Subsystem1/3(FAMLYRR3LFwdBkwdTrgtPosCalib_TrgtPosArray_write) -> FAMLYRR3LFwdBkwdTrgtPosCalib_TrgtPosArray_write/1
  Subsystem1/4(LugLR3LFwdBkwdTrgtPosCalib_TrgtPosArray_write) -> LugLR3LFwdBkwdTrgtPosCalib_TrgtPosArray_write/1
  Subsystem1/5(VIPR3LFwdBkwdTrgtPosCalib_TrgtPosArray_write) -> VIPR3LFwdBkwdTrgtPosCalib_TrgtPosArray_write/1
  Subsystem1/6(Md56R3LFwdBkwdTrgtPosCalib_TrgtPosArray_write) -> Md56R3LFwdBkwdTrgtPosCalib_TrgtPosArray_write/1
  Subsystem1/7(ThdRwLtStFwdBkwdEnTrigBitMask_Val_write) -> ThdRwLtStFwdBkwdEnTrigBitMask_Val_write/1
  Subsystem1/8(Md57R3LFwdBkwdTrgtPosCalib_TrgtPosArray) -> Md57R3LFwdBkwdTrgtPosCalib_TrgtPosArray/1
  Subsystem1/9(Md27R3LFwdBkwdTrgtPosCalib_TrgtPosArray_write) -> Md27R3LFwdBkwdTrgtPosCalib_TrgtPosArray_write/1

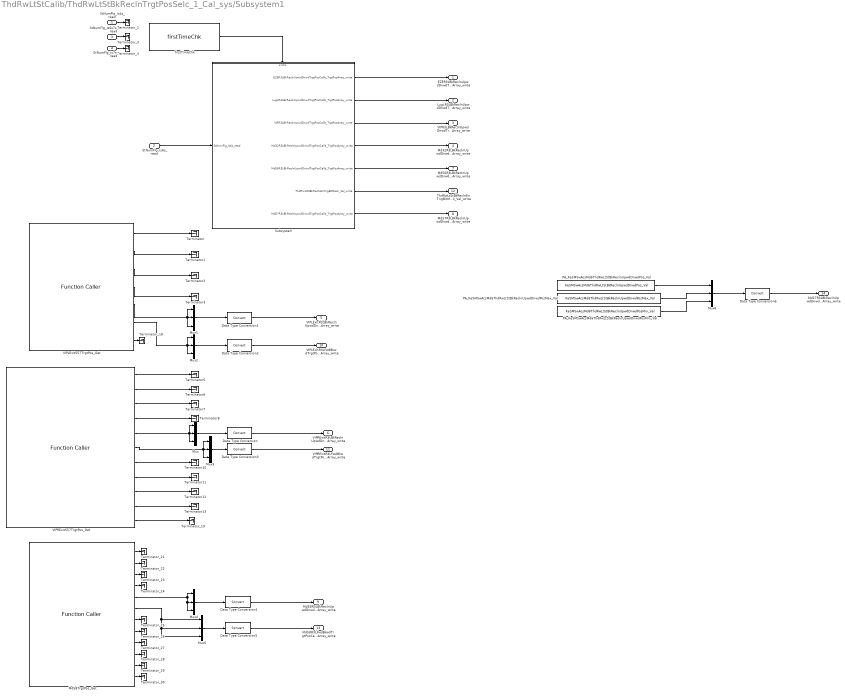
== system ThdRwLtStCalib/ThdRwLtStBkReclnTrgtPosSelc_1_Cal_sys/Subsystem1 ==
  StNumFlg_Is4s_read : Inport
  StNumFlg_Is6s_read : Inport  Port=2
  StNumFlg_Is6s7s_read : Inport  Port=3
  StNumFlg_Is7s_read : Inport  Port=4
  Data Type Conversion{,1..6} (7 alike) : DataTypeConversion  SaturateOnIntegerOverflow=off  RndMeth=Floor
  Md58TrgtPos_Get : FunctionCaller  FunctionPrototype=[SecRwRtStBkReclnTrgtPos,SecRwRtStZeroTrgtPos,SecRwRtStLgrstUpwdDnwdTrgtPos,SecRwRtStLgrstInwdOtwdTrgtPos,ThdRwLtStBkReclnTrgtPos,ThdRwLtStFwdBkwdTrgtPos,ThdRwRtStBkReclnTrgtPos,ThdRwRtStFwdBkwdTrgtPos,PassStBkReclnTrgtPos,PassStFwdBkwdTrgtPos,SecRwRtStFwdBkwdTrgtPos,PassStFldTrgtPos] = Md58TrgtPos_Get()  InputArgumentSpecifications=<Enter example>  OutputArgumentSpecifications=uint16(1), uint16(1), uint16(1), uint16(1), uint16(1), uint16(1), uint16(1), uint16(1), uint16(1), uint16(1), uint16(1), uint16(1)
  Mux{,1..6} (7 alike) : Mux  Inputs=3
  PA_KeSMSwAcsMd6ThdRwLtStBkReclnUpwdDnwdPosMax_Val : Constant  Value=KeSMSwAcsMd6ThdRwLtStBkReclnUpwdDnwdPosMax_Val
  PA_KeSMSwAcsMd6ThdRwLtStBkReclnUpwdDnwdPosMin_Val : Constant  Value=KeSMSwAcsMd6ThdRwLtStBkReclnUpwdDnwdPosMin_Val
  PA_KeSMSwAcsMd6ThdRwLtStBkReclnUpwdDnwdPos_Val : Constant  Value=KeSMSwAcsMd6ThdRwLtStBkReclnUpwdDnwdPos_Val
  Subsystem : Subsystem
  Terminator{,1..3,5..8,10..13} (12 alike) : Terminator
  Terminator_{1,3..4,18..19,21..30} (15 alike) : Terminator
  VIPLExit557TrgtPos_Get : FunctionCaller  FunctionPrototype=[SecRwLtStBkReclnTrgtPos,SecRwLtStZeroTrgtPos,SecRwLtStLgrstUpwdDnwdTrgtPos,SecRwLtStLgrstInwdOtwdTrgtPos,ThdRwLtStBkReclnTrgtPos,ThdRwLtStFwdBkwdTrgtPos,SecRwLtStFwdBkwdTrgtPos] = VIPLExit557TrgtPos_Get()  InputArgumentSpecifications=<Enter example>  OutputArgumentSpecifications=uint16(1), uint16(1), uint16(1), uint16(1), uint16(1), uint16(1), uint16(1)
  VIPRExit557TrgtPos_Get : FunctionCaller  FunctionPrototype=[SecRwRtStBkReclnTrgtPos,SecRwRtStZeroTrgtPos,SecRwRtStLgrstUpwdDnwdTrgtPos,SecRwRtStLgrstInwdOtwdTrgtPos,ThdRwLtStBkReclnTrgtPos,ThdRwLtStFwdBkwdTrgtPos,ThdRwRtStBkReclnTrgtPos,ThdRwRtStFwdBkwdTrgtPos,PassStBkReclnTrgtPos,PassStFwdBkwdTrgtPos,SecRwRtStFwdBkwdTrgtPos] = VIPRExit557TrgtPos_Get()  InputArgumentSpecifications=<Enter example>  OutputArgumentSpecifications=uint16(1), uint16(1), uint16(1), uint16(1), uint16(1), uint16(1), uint16(1), uint16(1), uint16(1), uint16(1), uint16(1)
  firstTimeChk : TrgtPosSelcLib/firstTimeChk  SystemSampleTime=-1  VariantActivationTime=update diagram  AllowFlexibleInterface=on  Latency=0  AutoFrameSizeCalculation=off
  EZER3LBkReclnUpwdDnwdTrgtPosCalib_TrgtPosArray_write : Outport  VectorParamsAs1DForOutWhenUnconnected=off
      settings: EnsureOutportIsVirtual=on
  LugLR3LBkReclnUpwdDnwdTrgtPosCalib_TrgtPosArray_write : Outport  Port=2  VectorParamsAs1DForOutWhenUnconnected=off
      settings: EnsureOutportIsVirtual=on
  VIPR3LBkReclnUpwdDnwdTrgtPosCalib_TrgtPosArray_write : Outport  Port=3  VectorParamsAs1DForOutWhenUnconnected=off
      settings: EnsureOutportIsVirtual=on
  Md32R3LBkReclnUpwdDnwdTrgtPosCalib_TrgtPosArray_write : Outport  Port=4  VectorParamsAs1DForOutWhenUnconnected=off
      settings: EnsureOutportIsVirtual=on
  VIPLExitR3LBkReclnUpwdDnwdTrgtPosCalib_TrgtPosArray_write : Outport  Port=5  VectorParamsAs1DForOutWhenUnconnected=off
      settings: EnsureOutportIsVirtual=on
  VIPRExitR3LBkReclnUpwdDnwdTrgtPosCalib_TrgtPosArray_write : Outport  Port=6  VectorParamsAs1DForOutWhenUnconnected=off
      settings: EnsureOutportIsVirtual=on
  Md56R3LBkReclnUpwdDnwdTrgtPosCalib_TrgtPosArray_write : Outport  Port=7  VectorParamsAs1DForOutWhenUnconnected=off
      settings: EnsureOutportIsVirtual=on
  Md57R3LBkReclnUpwdDnwdTrgtPosCalib_TrgtPosArray_write : Outport  Port=8  VectorParamsAs1DForOutWhenUnconnected=off
      settings: EnsureOutportIsVirtual=on
  Md58R3LBkReclnUpwdDnwdTrgtPosCalib_TrgtPosArray_write : Outport  Port=9  VectorParamsAs1DForOutWhenUnconnected=off
      settings: EnsureOutportIsVirtual=on
  VIPLExitR3LFwdBkwdTrgtPosCalib_TrgtPosArray_write : Outport  Port=10  VectorParamsAs1DForOutWhenUnconnected=off
      settings: EnsureOutportIsVirtual=on
  VIPRExitR3LFwdBkwdTrgtPosCalib_TrgtPosArray_write : Outport  Port=11  VectorParamsAs1DForOutWhenUnconnected=off
      settings: EnsureOutportIsVirtual=on
  ThdRwLtStBkReclnEnTrigBitMask_Val_write : Outport  Port=12  VectorParamsAs1DForOutWhenUnconnected=off
      settings: EnsureOutportIsVirtual=on
  Md58R3LFwdBkwdTrgtPosCalib_TrgtPosArray_write : Outport  Port=13  VectorParamsAs1DForOutWhenUnconnected=off
      settings: EnsureOutportIsVirtual=on
  Md27R3LBkReclnUpwdDnwdTrgtPosCalib_TrgtPosArray_write : Outport  Port=14  VectorParamsAs1DForOutWhenUnconnected=off
  wires:
  StNumFlg_Is6s7s_read/1 -> Terminator_3/1
  StNumFlg_Is4s_read/1 -> Terminator_1/1
  StNumFlg_Is6s_read/1 -> Subsystem/1(StNumFlg_Is6s_read)
  Subsystem/2(LugLR3LBkReclnUpwdDnwdTrgtPosCalib_TrgtPosArray_write) -> LugLR3LBkReclnUpwdDnwdTrgtPosCalib_TrgtPosArray_write/1
  firstTimeChk/1 -> Subsystem/Enable
  StNumFlg_Is7s_read/1 -> Terminator_4/1
  Subsystem/3(VIPR3LBkReclnUpwdDnwdTrgtPosCalib_TrgtPosArray_write) -> VIPR3LBkReclnUpwdDnwdTrgtPosCalib_TrgtPosArray_write/1
  Subsystem/1(EZER3LBkReclnUpwdDnwdTrgtPosCalib_TrgtPosArray_write) -> EZER3LBkReclnUpwdDnwdTrgtPosCalib_TrgtPosArray_write/1
  Subsystem/4(Md32R3LBkReclnUpwdDnwdTrgtPosCalib_TrgtPosArray_write) -> Md32R3LBkReclnUpwdDnwdTrgtPosCalib_TrgtPosArray_write/1
  VIPRExit557TrgtPos_Get/5 -> Mux/1, Mux/3, Mux/2
  Mux/1 -> Data Type Conversion/1
  Data Type Conversion/1 -> VIPRExitR3LBkReclnUpwdDnwdTrgtPosCalib_TrgtPosArray_write/1
  Data Type Conversion1/1 -> VIPLExitR3LBkReclnUpwdDnwdTrgtPosCalib_TrgtPosArray_write/1
  Mux1/1 -> Data Type Conversion1/1
  VIPLExit557TrgtPos_Get/5 -> Mux1/1, Mux1/2, Mux1/3
  VIPLExit557TrgtPos_Get/1 -> Terminator/1
  VIPLExit557TrgtPos_Get/2 -> Terminator1/1
  VIPLExit557TrgtPos_Get/3 -> Terminator2/1
  VIPLExit557TrgtPos_Get/4 -> Terminator3/1
  VIPRExit557TrgtPos_Get/1 -> Terminator5/1
  VIPRExit557TrgtPos_Get/2 -> Terminator6/1
  VIPRExit557TrgtPos_Get/3 -> Terminator7/1
  VIPRExit557TrgtPos_Get/4 -> Terminator8/1
  VIPRExit557TrgtPos_Get/7 -> Terminator10/1
  VIPRExit557TrgtPos_Get/8 -> Terminator11/1
  VIPRExit557TrgtPos_Get/9 -> Terminator12/1
  VIPRExit557TrgtPos_Get/10 -> Terminator13/1
  VIPLExit557TrgtPos_Get/7 -> Terminator_18/1
  VIPRExit557TrgtPos_Get/11 -> Terminator_19/1
  Subsystem/5(Md56R3LBkReclnUpwdDnwdTrgtPosCalib_TrgtPosArray_write) -> Md56R3LBkReclnUpwdDnwdTrgtPosCalib_TrgtPosArray_write/1
  VIPLExit557TrgtPos_Get/6 -> Mux2/3, Mux2/2, Mux2/1
  Mux2/1 -> Data Type Conversion2/1
  Data Type Conversion2/1 -> VIPLExitR3LFwdBkwdTrgtPosCalib_TrgtPosArray_write/1
  Data Type Conversion3/1 -> VIPRExitR3LFwdBkwdTrgtPosCalib_TrgtPosArray_write/1
  Mux3/1 -> Data Type Conversion3/1
  VIPRExit557TrgtPos_Get/6 -> Mux3/2, Mux3/3, Mux3/1
  Subsystem/6(ThdRwLtStBkReclnEnTrigBitMask_Val_write) -> ThdRwLtStBkReclnEnTrigBitMask_Val_write/1
  Subsystem/7(Md57R3LBkReclnUpwdDnwdTrgtPosCalib_TrgtPosArray_write) -> Md57R3LBkReclnUpwdDnwdTrgtPosCalib_TrgtPosArray_write/1
  Data Type Conversion4/1 -> Md58R3LBkReclnUpwdDnwdTrgtPosCalib_TrgtPosArray_write/1
  Mux4/1 -> Data Type Conversion4/1
  Md58TrgtPos_Get/5 -> Mux4/2, Mux4/3, Mux4/1
  Md58TrgtPos_Get/6 -> Mux5/3, Mux5/2, Mux5/1
  Mux5/1 -> Data Type Conversion5/1
  Data Type Conversion5/1 -> Md58R3LFwdBkwdTrgtPosCalib_TrgtPosArray_write/1
  Md58TrgtPos_Get/1 -> Terminator_21/1
  Md58TrgtPos_Get/2 -> Terminator_22/1
  Md58TrgtPos_Get/3 -> Terminator_23/1
  Md58TrgtPos_Get/4 -> Terminator_24/1
  Md58TrgtPos_Get/7 -> Terminator_25/1
  Md58TrgtPos_Get/8 -> Terminator_26/1
  Md58TrgtPos_Get/9 -> Terminator_27/1
  Md58TrgtPos_Get/10 -> Terminator_28/1
  Md58TrgtPos_Get/11 -> Terminator_29/1
  Md58TrgtPos_Get/12 -> Terminator_30/1
  Mux6/1 -> Data Type Conversion6/1
  Data Type Conversion6/1 -> Md27R3LBkReclnUpwdDnwdTrgtPosCalib_TrgtPosArray_write/1
  PA_KeSMSwAcsMd6ThdRwLtStBkReclnUpwdDnwdPos_Val/1 -> Mux6/1
  PA_KeSMSwAcsMd6ThdRwLtStBkReclnUpwdDnwdPosMax_Val/1 -> Mux6/2
  PA_KeSMSwAcsMd6ThdRwLtStBkReclnUpwdDnwdPosMin_Val/1 -> Mux6/3

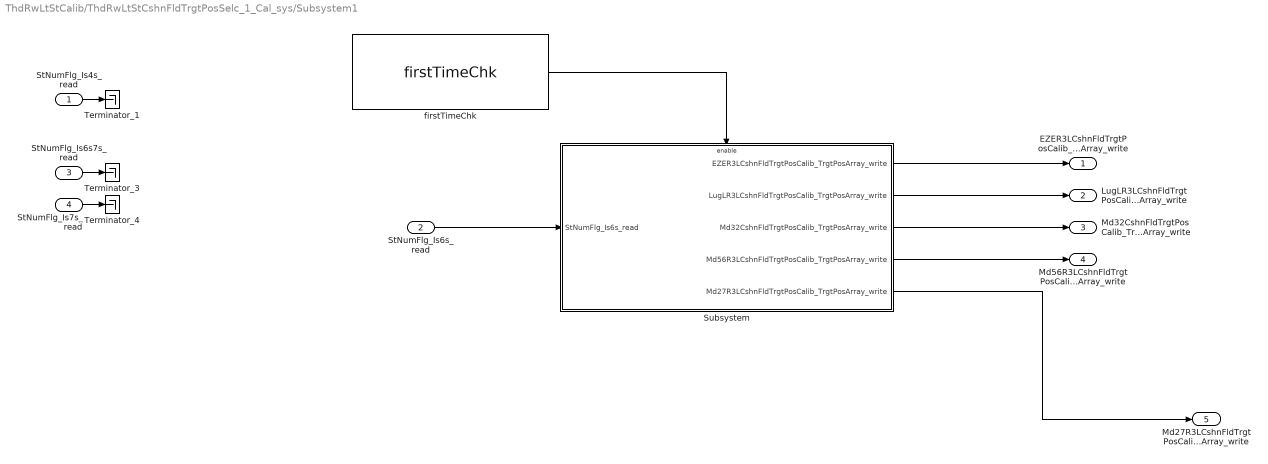
== system ThdRwLtStCalib/ThdRwLtStCshnFldTrgtPosSelc_1_Cal_sys/Subsystem1 ==
  StNumFlg_Is4s_read : Inport
  StNumFlg_Is6s_read : Inport  Port=2
  StNumFlg_Is6s7s_read : Inport  Port=3
  StNumFlg_Is7s_read : Inport  Port=4
  Subsystem : Subsystem
  Terminator_1 : Terminator
  Terminator_3 : Terminator
  Terminator_4 : Terminator
  firstTimeChk : TrgtPosSelcLib/firstTimeChk  SystemSampleTime=-1  VariantActivationTime=update diagram  AllowFlexibleInterface=on  Latency=0  AutoFrameSizeCalculation=off
  EZER3LCshnFldTrgtPosCalib_TrgtPosArray_write : Outport  VectorParamsAs1DForOutWhenUnconnected=off
      settings: EnsureOutportIsVirtual=on
  LugLR3LCshnFldTrgtPosCalib_TrgtPosArray_write : Outport  Port=2  VectorParamsAs1DForOutWhenUnconnected=off
      settings: EnsureOutportIsVirtual=on
  Md32CshnFldTrgtPosCalib_TrgtPosArray_write : Outport  Port=3  VectorParamsAs1DForOutWhenUnconnected=off
      settings: EnsureOutportIsVirtual=on
  Md56R3LCshnFldTrgtPosCalib_TrgtPosArray_write : Outport  Port=4  VectorParamsAs1DForOutWhenUnconnected=off
      settings: EnsureOutportIsVirtual=on
  Md27R3LCshnFldTrgtPosCalib_TrgtPosArray_write : Outport  Port=5  VectorParamsAs1DForOutWhenUnconnected=off
  wires:
  StNumFlg_Is4s_read/1 -> Terminator_1/1
  StNumFlg_Is7s_read/1 -> Terminator_4/1
  StNumFlg_Is6s7s_read/1 -> Terminator_3/1
  StNumFlg_Is6s_read/1 -> Subsystem/1(StNumFlg_Is6s_read)
  firstTimeChk/1 -> Subsystem/Enable
  Subsystem/1(EZER3LCshnFldTrgtPosCalib_TrgtPosArray_write) -> EZER3LCshnFldTrgtPosCalib_TrgtPosArray_write/1
  Subsystem/2(LugLR3LCshnFldTrgtPosCalib_TrgtPosArray_write) -> LugLR3LCshnFldTrgtPosCalib_TrgtPosArray_write/1
  Subsystem/3(Md32CshnFldTrgtPosCalib_TrgtPosArray_write) -> Md32CshnFldTrgtPosCalib_TrgtPosArray_write/1
  Subsystem/4(Md56R3LCshnFldTrgtPosCalib_TrgtPosArray_write) -> Md56R3LCshnFldTrgtPosCalib_TrgtPosArray_write/1
  Subsystem/5(Md27R3LCshnFldTrgtPosCalib_TrgtPosArray_write) -> Md27R3LCshnFldTrgtPosCalib_TrgtPosArray_write/1

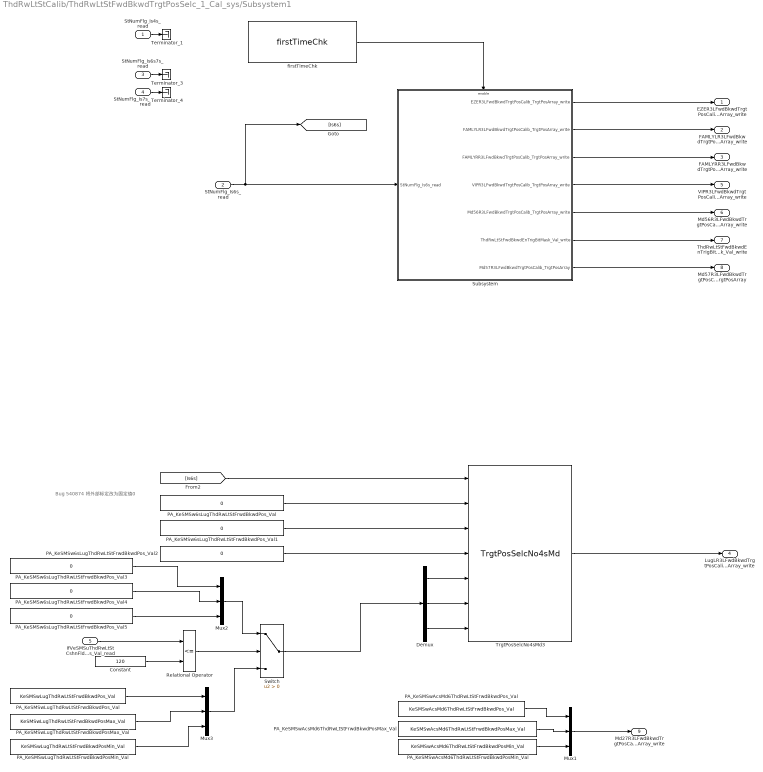
== system ThdRwLtStCalib/ThdRwLtStFwdBkwdTrgtPosSelc_1_Cal_sys/Subsystem1 ==
  note: Bug 540874 将外部标定改为固定值0
  StNumFlg_Is4s_read : Inport
  StNumFlg_Is6s_read : Inport  Port=2
  StNumFlg_Is6s7s_read : Inport  Port=3
  StNumFlg_Is7s_read : Inport  Port=4
  IfVeSMSuThdRwLtStCshnFldUpwdDnwdPos_Val_read : Inport  Port=5
  Constant : Constant  Value=120  OutDataTypeStr=uint16
  Demux : Demux  Outputs=3
  Mux1 : Mux  Inputs=3
  Mux2 : Mux  Inputs=3
  Mux3 : Mux  Inputs=3
  PA_KeSMSw6sLugThdRwLtStFrwdBkwdPos_Val{,1..5} (6 alike) : Constant  Value=0  OutDataTypeStr=uint16
  PA_KeSMSwAcsMd6ThdRwLtStFrwdBkwdPosMax_Val : Constant  Value=KeSMSwAcsMd6ThdRwLtStFrwdBkwdPosMax_Val
  PA_KeSMSwAcsMd6ThdRwLtStFrwdBkwdPosMin_Val : Constant  Value=KeSMSwAcsMd6ThdRwLtStFrwdBkwdPosMin_Val
  PA_KeSMSwAcsMd6ThdRwLtStFrwdBkwdPos_Val : Constant  Value=KeSMSwAcsMd6ThdRwLtStFrwdBkwdPos_Val
  PA_KeSMSwLugThdRwLtStFrwdBkwdPosMax_Val : Constant  Value=KeSMSwLugThdRwLtStFrwdBkwdPosMax_Val
  PA_KeSMSwLugThdRwLtStFrwdBkwdPosMin_Val : Constant  Value=KeSMSwLugThdRwLtStFrwdBkwdPosMin_Val
  PA_KeSMSwLugThdRwLtStFrwdBkwdPos_Val : Constant  Value=KeSMSwLugThdRwLtStFrwdBkwdPos_Val
  Relational Operator : RelationalOperator  Operator=<=  OutDataTypeStr=boolean  RndMeth=Simplest  InputSameDT=off
  Subsystem : Subsystem
  Switch : Switch  Criteria=u2 > Threshold  SaturateOnIntegerOverflow=off  InputSameDT=off
  Terminator_1 : Terminator
  Terminator_3 : Terminator
  Terminator_4 : Terminator
  TrgtPosSelcNo4sMd3 : TrgtPosSelcLib/TrgtPosSelcNo4sMd  SystemSampleTime=-1  VariantActivationTime=update diagram  AllowFlexibleInterface=on  Latency=0  AutoFrameSizeCalculation=off
  firstTimeChk : TrgtPosSelcLib/firstTimeChk  SystemSampleTime=-1  VariantActivationTime=update diagram  AllowFlexibleInterface=on  Latency=0  AutoFrameSizeCalculation=off
  EZER3LFwdBkwdTrgtPosCalib_TrgtPosArray_write : Outport  VectorParamsAs1DForOutWhenUnconnected=off
      settings: EnsureOutportIsVirtual=on
  FAMLYLR3LFwdBkwdTrgtPosCalib_TrgtPosArray_write : Outport  Port=2  VectorParamsAs1DForOutWhenUnconnected=off
      settings: EnsureOutportIsVirtual=on
  FAMLYRR3LFwdBkwdTrgtPosCalib_TrgtPosArray_write : Outport  Port=3  VectorParamsAs1DForOutWhenUnconnected=off
      settings: EnsureOutportIsVirtual=on
  LugLR3LFwdBkwdTrgtPosCalib_TrgtPosArray_write : Outport  Port=4  VectorParamsAs1DForOutWhenUnconnected=off
      settings: EnsureOutportIsVirtual=on
  VIPR3LFwdBkwdTrgtPosCalib_TrgtPosArray_write : Outport  Port=5  VectorParamsAs1DForOutWhenUnconnected=off
      settings: EnsureOutportIsVirtual=on
  Md56R3LFwdBkwdTrgtPosCalib_TrgtPosArray_write : Outport  Port=6  VectorParamsAs1DForOutWhenUnconnected=off
      settings: EnsureOutportIsVirtual=on
  ThdRwLtStFwdBkwdEnTrigBitMask_Val_write : Outport  Port=7  VectorParamsAs1DForOutWhenUnconnected=off
      settings: EnsureOutportIsVirtual=on
  Md57R3LFwdBkwdTrgtPosCalib_TrgtPosArray : Outport  Description=|  Port=8  OutDataTypeStr=uint16  PortDimensions=3  VectorParamsAs1DForOutWhenUnconnected=off
      | 0:Pos
      | 1:Max
      | 2:Min
  Md27R3LFwdBkwdTrgtPosCalib_TrgtPosArray_write : Outport  Port=9  VectorParamsAs1DForOutWhenUnconnected=off
  wires:
  Subsystem/4(VIPR3LFwdBkwdTrgtPosCalib_TrgtPosArray_write) -> VIPR3LFwdBkwdTrgtPosCalib_TrgtPosArray_write/1
  StNumFlg_Is7s_read/1 -> Terminator_4/1
  TrgtPosSelcNo4sMd3/1 -> LugLR3LFwdBkwdTrgtPosCalib_TrgtPosArray_write/1
  StNumFlg_Is4s_read/1 -> Terminator_1/1
  Subsystem/2(FAMLYLR3LFwdBkwdTrgtPosCalib_TrgtPosArray_write) -> FAMLYLR3LFwdBkwdTrgtPosCalib_TrgtPosArray_write/1
  Subsystem/3(FAMLYRR3LFwdBkwdTrgtPosCalib_TrgtPosArray_write) -> FAMLYRR3LFwdBkwdTrgtPosCalib_TrgtPosArray_write/1
  Subsystem/1(EZER3LFwdBkwdTrgtPosCalib_TrgtPosArray_write) -> EZER3LFwdBkwdTrgtPosCalib_TrgtPosArray_write/1
  firstTimeChk/1 -> Subsystem/Enable
  StNumFlg_Is6s_read/1 -> [Is6s], Subsystem/1(StNumFlg_Is6s_read)
  StNumFlg_Is6s7s_read/1 -> Terminator_3/1
  PA_KeSMSw6sLugThdRwLtStFrwdBkwdPos_Val2/1 -> TrgtPosSelcNo4sMd3/4
  PA_KeSMSw6sLugThdRwLtStFrwdBkwdPos_Val1/1 -> TrgtPosSelcNo4sMd3/3
  PA_KeSMSw6sLugThdRwLtStFrwdBkwdPos_Val/1 -> TrgtPosSelcNo4sMd3/2
  [Is6s] -> TrgtPosSelcNo4sMd3/1
  IfVeSMSuThdRwLtStCshnFldUpwdDnwdPos_Val_read/1 -> Relational Operator/1
  Constant/1 -> Relational Operator/2
  Relational Operator/1 -> Switch/2
  Mux2/1 -> Switch/1
  PA_KeSMSw6sLugThdRwLtStFrwdBkwdPos_Val3/1 -> Mux2/1
  PA_KeSMSw6sLugThdRwLtStFrwdBkwdPos_Val4/1 -> Mux2/2
  PA_KeSMSw6sLugThdRwLtStFrwdBkwdPos_Val5/1 -> Mux2/3
  PA_KeSMSwLugThdRwLtStFrwdBkwdPos_Val/1 -> Mux3/1
  PA_KeSMSwLugThdRwLtStFrwdBkwdPosMax_Val/1 -> Mux3/2
  PA_KeSMSwLugThdRwLtStFrwdBkwdPosMin_Val/1 -> Mux3/3
  Mux3/1 -> Switch/3
  Switch/1 -> Demux/1
  Demux/1 -> TrgtPosSelcNo4sMd3/5
  Demux/2 -> TrgtPosSelcNo4sMd3/6
  Demux/3 -> TrgtPosSelcNo4sMd3/7
  Subsystem/5(Md56R3LFwdBkwdTrgtPosCalib_TrgtPosArray_write) -> Md56R3LFwdBkwdTrgtPosCalib_TrgtPosArray_write/1
  Subsystem/6(ThdRwLtStFwdBkwdEnTrigBitMask_Val_write) -> ThdRwLtStFwdBkwdEnTrigBitMask_Val_write/1
  Subsystem/7(Md57R3LFwdBkwdTrgtPosCalib_TrgtPosArray) -> Md57R3LFwdBkwdTrgtPosCalib_TrgtPosArray/1
  Mux1/1 -> Md27R3LFwdBkwdTrgtPosCalib_TrgtPosArray_write/1
  PA_KeSMSwAcsMd6ThdRwLtStFrwdBkwdPosMin_Val/1 -> Mux1/3
  PA_KeSMSwAcsMd6ThdRwLtStFrwdBkwdPosMax_Val/1 -> Mux1/2
  PA_KeSMSwAcsMd6ThdRwLtStFrwdBkwdPos_Val/1 -> Mux1/1
